simulink model "Que1"  (R2023b)
settings: Solver=VariableStepAuto  StartTime=0.0  StopTime=30.0  RelTol=1e-3
settings Model: Creator=setak  LastModifiedBy=setak

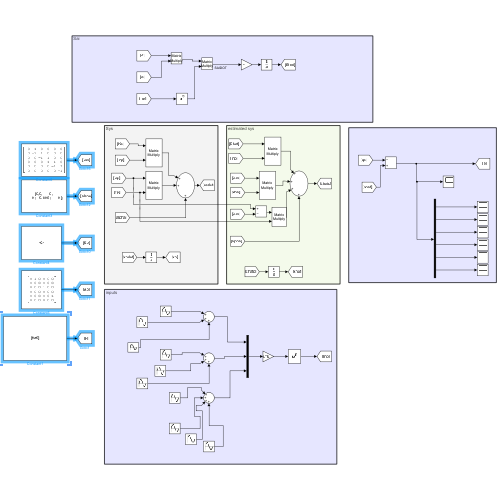
[thumbnail: Simulink's stored preview of the top-level diagram]
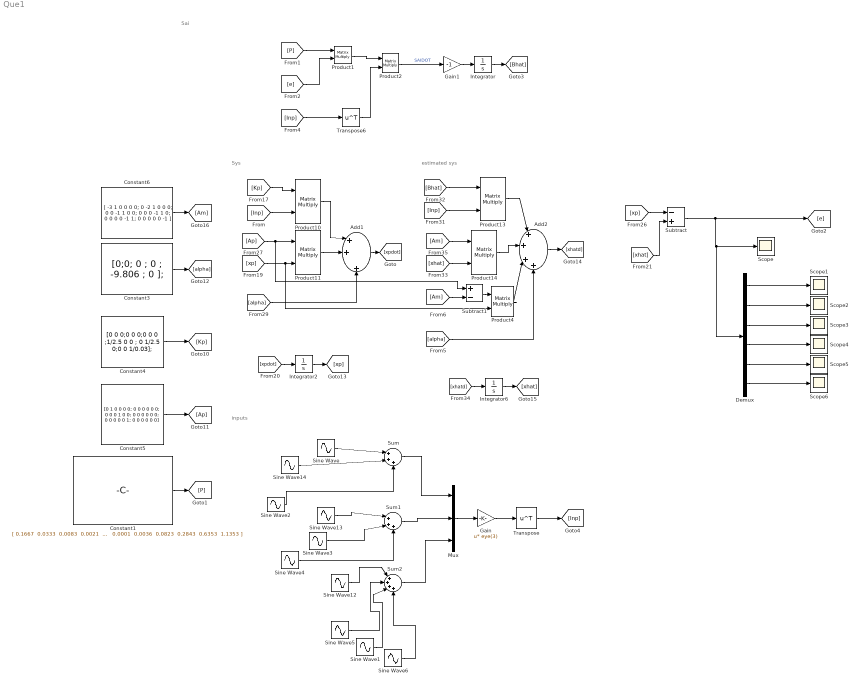
== system Que1 ==
  note: inputs
  note: estimated sys
  note: Sys
  note: Sai
  Add1 : Sum  Inputs=|++|+
  Add2 : Sum  Inputs=|+|+|+|+
  Constant1 : Constant  Value=|
      | [ 0.1667  0.0333  0.0083  0.0021  0.0005  0.0001;
      |           0.0333  0.2667  0.0917  0.0312  0.0106  0.0036;
      |           0.0083  0.0917  0.5917  0.3115  0.1610  0.0823;
      |           0.0021  0.0312  0.3115  0.8115  0.4862  0.2843;
      |           0.0005  0.0106  0.1610  0.4862  0.9862  0.6353;
      |           0.0001  0.0036  0.0823  0.2843  0.6353  1.1353 ]
  Constant3 : Constant  Value=|
      | [0;0;      0 ;
      |       0 ;  -9.806 ;      0 ];
  Constant4 : Constant  Value="[0 0 0;0 0 0;0 0 0 ;1/2.5 0 0  ; 0 1/2.5  0;0 0 1/0.03];"
  Constant5 : Constant  Value=|
      | [0 1 0 0 0 0;      0 0 0 0 0 0;
      |       0 0 0 1 0 0;      0 0 0 0 0 0;
      |       0 0 0 0 0 1;      0 0 0 0 0 0]
  Constant6 : Constant  Value=|
      | [ -3  1  0  0  0  0;
      |             0 -2  1  0  0  0;
      |             0  0 -1  1  0  0;
      |             0  0  0 -1  1  0;
      |             0  0  0  0 -1  1;
      |             0  0  0  0  0 -1 ]
  Demux : Demux  Outputs=6
  Gain : Gain  Gain=eye(3)  Multiplication=Matrix(u*K)
  Gain1 : Gain  Gain=-1
  Integrator : Integrator
  Integrator2 : Integrator  InitialCondition=[0 ;0; 0;0;0;0]
  Integrator6 : Integrator  InitialCondition=[0; 0; 0;0;0;0]
  Mux : Mux  Inputs=3
  Product{1..2,4,10..11,13..14} (7 alike) : Product  Multiplication=Matrix(*)
  Scope{,1..6} (7 alike) : Scope
  Sine Wave : Sin  SampleTime=0
  Sine Wave1 : Sin  Amplitude=9  Frequency=9  SampleTime=0
  Sine Wave12 : Sin  Amplitude=7  Frequency=7  SampleTime=0
  Sine Wave13 : Sin  Frequency=4  SampleTime=0
  Sine Wave14 : Sin  Frequency=2  SampleTime=0
  Sine Wave2 : Sin  Amplitude=2  Frequency=3  SampleTime=0
  Sine Wave3 : Sin  Amplitude=3  Frequency=5  SampleTime=0
  Sine Wave4 : Sin  Amplitude=6  Frequency=6  SampleTime=0
  Sine Wave5 : Sin  Amplitude=8  Frequency=8  SampleTime=0
  Sine Wave6 : Sin  Amplitude=10  Frequency=10  SampleTime=0
  Subtract : Sum  Inputs=-+
  Subtract1 : Sum  Inputs=+-
  Sum : Sum  Inputs=|+++
  Sum1 : Sum  Inputs=|+++
  Sum2 : Sum  Inputs=|++++
  Transpose : Math  Operator=transpose
  Transpose6 : Math  Operator=transpose
  wires:
  Product14/1 -> Add2/2
  Transpose/1 -> [Inp]
  Add1/1 -> [xpdot]
  Product2/1 -> Gain1/1  "SAIDOT"
  Sine Wave12/1 -> Sum2/1
  Transpose6/1 -> Product2/2
  Constant4/1 -> [Kp]
  [Inp] -> Transpose6/1
  Sine Wave14/1 -> Sum/2
  Product13/1 -> Add2/1
  Sine Wave4/1 -> Sum1/3
  Constant1/1 -> [P]
  Sine Wave/1 -> Sum/1
  [alpha] -> Add1/3
  Mux/1 -> Gain/1
  Sine Wave13/1 -> Sum1/1
  Product1/1 -> Product2/1
  [Am] -> Product14/1
  Sum2/1 -> Mux/3
  [P] -> Product1/1
  Sine Wave5/1 -> Sum2/2
  [xp] -> Product4/2, Product11/2
  [xhatd] -> Integrator6/1
  Sine Wave3/1 -> Sum1/2
  Sum/1 -> Mux/1
  Product11/1 -> Add1/2
  Subtract/1 -> Demux/1, Scope/1, [e]
  Constant3/1 -> [alpha]
  Integrator/1 -> [Bhat]
  Gain1/1 -> Integrator/1
  [Bhat] -> Product13/1
  [e] -> Product1/2
  Constant5/1 -> [Ap]
  [xhat] -> Product14/2
  Integrator6/1 -> [xhat]
  [Inp] -> Product10/2
  Integrator2/1 -> [xp]
  [Ap] -> Subtract1/1, Product11/1
  [xp] -> Subtract/1
  [Inp] -> Product13/2
  [xhat] -> Subtract/2
  Product10/1 -> Add1/1
  Sum1/1 -> Mux/2
  Add2/1 -> [xhatd]
  [xpdot] -> Integrator2/1
  [Kp] -> Product10/1
  Gain/1 -> Transpose/1
  Demux/1 -> Scope1/1
  Demux/2 -> Scope2/1
  Demux/3 -> Scope3/1
  Demux/4 -> Scope4/1
  Demux/5 -> Scope5/1
  Demux/6 -> Scope6/1
  [alpha] -> Add2/4
  Sine Wave2/1 -> Sum/3
  [Am] -> Subtract1/2
  Subtract1/1 -> Product4/1
  Constant6/1 -> [Am]
  Sine Wave1/1 -> Sum2/3
  Sine Wave6/1 -> Sum2/4
  Product4/1 -> Add2/3
